simulink model "testbench_sensor"  (R2015a)
settings: Solver=ode3  StartTime=0.0  StopTime=10.0  RelTol=1e-3
libraries: legoev3lib x3, simulink x1
settings Model: SimulationMode=external  ExtModeTrigDuration=2  Creator=G. Eranna  LastModifiedBy=USER
settings OptimizationCC: OptimizeModelRefInitCode=on  LifeSpan=1
settings DebuggingCC: UnderspecifiedInitializationDetection=Classic  MergeDetectMultiDrivingBlocksExec=none
settings HardwareCC: ProdLargestAtomicInteger=Long  ProdLargestAtomicFloat=Float  ProdEndianess=LittleEndian  ProdHWDeviceType=ARM Compatible->ARM 9
settings RTWCC: SystemTargetFile=realtime.tlc  GenerateMakefile=off  TemplateMakefile=realtime.tmf  Description=Run on Target Hardware  RTWVerbose=off
settings ERTTargetCC: CombineOutputUpdateFcns=off  ERTSrcFileBannerTemplate=realtime_code_template.cgt  ERTHdrFileBannerTemplate=realtime_code_template.cgt  ERTDataSrcFileTemplate=realtime_code_template.cgt  ERTDataHdrFileTemplate=realtime_code_template.cgt  ERTCustomFileTemplate=realtime_file_process.tlc

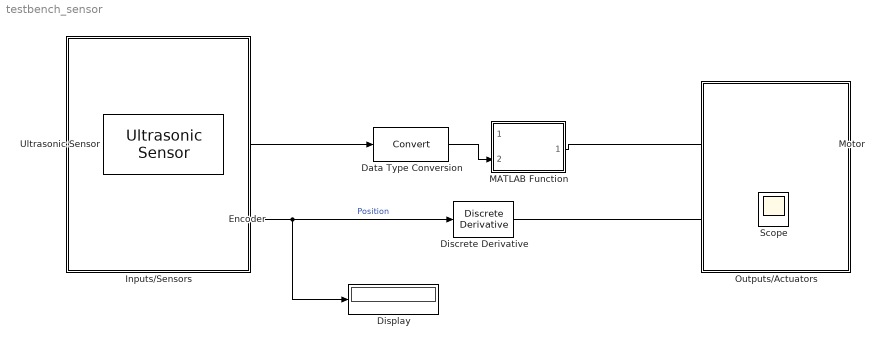
== system testbench_sensor ==
  Data Type Conversion : DataTypeConversion
  Discrete Derivative : simulink/Discrete/Discrete Derivative  gainval=1.0  ICPrevScaledInput=800  InputProcessing=Inherited  OutMin=[]  OutMax=[]  OutDataTypeStr=double  OutputDataTypeScalingMode=double  OutDataType=fixdt(1, 16)  OutScaling=2^-10  DoSatur=off
  Display : Display
  Encoder : legoev3lib/Encoder  portNumber=A  opMode=No reset  sampleTime=0.01
  Inputs/Sensors : Subsystem
  MATLAB Function : MATLAB Function  TreatAsAtomicUnit=on
  Motor : legoev3lib/Motor  sportNumber=A  sstopAction=Brake
  Outputs/Actuators : Subsystem
  Scope : Scope  NumInputPorts=3
      settings: YMin=-90~-1000~100  YMax=80~1000~800  SaveName=acqData
  Ultrasonic Sensor : legoev3lib/Ultrasonic Sensor  PortNumber=1  sampleTime=0.1
  wires:
  Data Type Conversion/1 -> MATLAB Function/2(sensor_input)
  MATLAB Function/1(rearmotor) -> Motor/1
  Encoder/1 -> Discrete Derivative/1, Display/1  "Position"
  Ultrasonic Sensor/1 -> Data Type Conversion/1
  Discrete Derivative/1 -> Scope/3

== system testbench_sensor/Inputs//Sensors ==

== system testbench_sensor/Outputs//Actuators ==

== matlab function testbench_sensor/MATLAB Function ==
  data: motor_input input; sensor_input input; rearmotor output
function rearmotor = fcn(motor_input,sensor_input)
%#codegen
if(sensor_input>4)&&(sensor_input<=20)
    rearmotor=motor_input;
%elseif(u>20)&&(u<=35)
 %   rearmotor=50;
else
    rearmotor=0;
end
end
